simulink library "chy_framelib"  (R2016a)
settings: Solver=ode1  StartTime=0.0  StopTime=Inf  FixedStep=0.001  RelTol=1e-3
undefined symbols (not defined in the file): emot_Ri_Inv
libraries: Powernet x1, Energy_converter_Electrical_to_Mechanical x1
settings Model: Creator=ASRANJA  LastModifiedBy=KNWINDE
settings DataIOCC: LimitDataPoints=on  SaveFormat=Array  SignalLoggingSaveFormat=ModelDataLogs
settings OptimizationCC: BlockReduction=off  OptimizeBlockIOStorage=off  BufferReuse=off  GlobalBufferReuse=off  ExpressionFolding=off  ExpressionDepthLimit=2147483647  LocalBlockOutputs=off
settings DebuggingCC: UnderspecifiedInitializationDetection=Classic  MergeDetectMultiDrivingBlocksExec=none  SolverPrmCheckMsg=warning  MultiTaskDSMMsg=warning  MultiTaskCondExecSysMsg=none  StateNameClashWarn=warning  StrictBusMsg=None
settings HardwareCC: ProdBitPerPointer=32  ProdLargestAtomicFloat=None  ProdIntDivRoundTo=Undefined  ProdEndianess=Unspecified  ProdWordSize=32  ProdHWDeviceType=32-bit Generic
settings ModelReferenceCC: PropagateSignalLabelsOutOfModel=off
settings RTWCC: SystemTargetFile=rti1401.tlc  MakeCommand=make_rti  TemplateMakefile=rti1401.tmf  Description=dSPACE DS1401 Hardware Platform
settings STFCustomTargetCC: ModelReferenceCompliant=off  GeneratePreprocessorConditionals=Disable all  CombineOutputUpdateFcns=on  MatFileLogging=on  MATLABClassNameForMDSCustomization=Simulink.SoftwareTarget.TargetSpecificTriggerConfigurationBase  CPPClassGenCompliant=on  GRTInterface=off  SystemTargetFile=rti1401.tlc
settings ConfigComp: CovModelRefEnable=Off

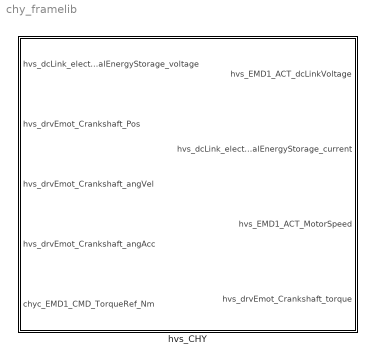
== system chy_framelib ==
  hvs_CHY : Subsystem

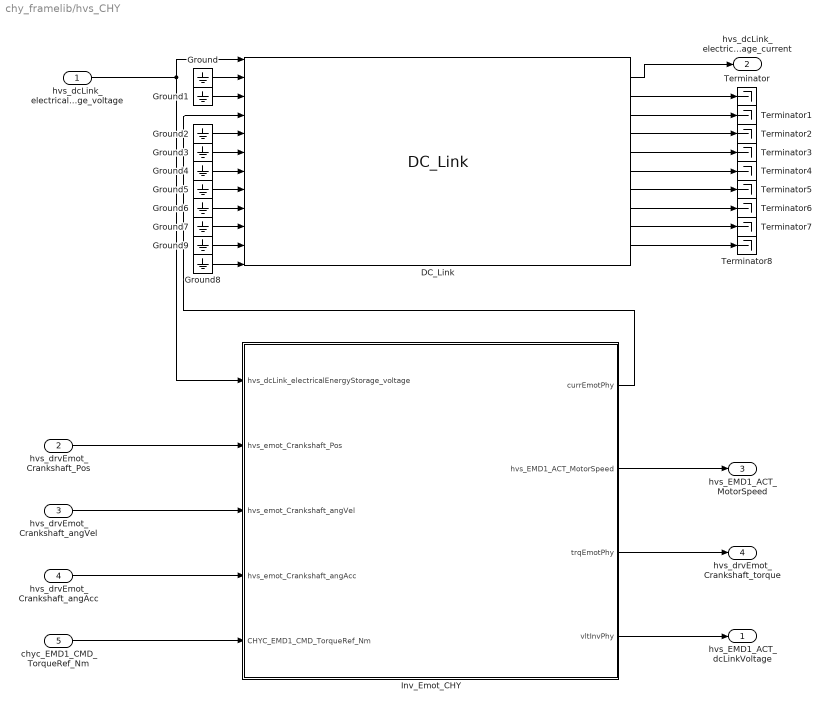
== system chy_framelib/hvs_CHY ==
  hvs_dcLink_electricalEnergyStorage_voltage : Inport
  hvs_drvEmot_Crankshaft_Pos : Inport  Port=2
  hvs_drvEmot_Crankshaft_angVel : Inport  Port=3
  hvs_drvEmot_Crankshaft_angAcc : Inport  Port=4
  chyc_EMD1_CMD_TorqueRef_Nm : Inport  Port=5
  DC_Link : Powernet/DC_Link
  Ground{,1..9} (10 alike) : Ground
  Inv_Emot_CHY : Subsystem
  Terminator{,1..8} (9 alike) : Terminator
  hvs_EMD1_ACT_dcLinkVoltage : Outport
  hvs_dcLink_electricalEnergyStorage_current : Outport  Port=2
  hvs_EMD1_ACT_MotorSpeed : Outport  Port=3
  hvs_drvEmot_Crankshaft_torque : Outport  Port=4
  wires:
  Inv_Emot_CHY/4(vltInvPhy) -> hvs_EMD1_ACT_dcLinkVoltage/1
  hvs_dcLink_electricalEnergyStorage_voltage/1 -> DC_Link/1, Inv_Emot_CHY/1(hvs_dcLink_electricalEnergyStorage_voltage)
  DC_Link/1 -> hvs_dcLink_electricalEnergyStorage_current/1
  hvs_drvEmot_Crankshaft_Pos/1 -> Inv_Emot_CHY/2(hvs_emot_Crankshaft_Pos)
  hvs_drvEmot_Crankshaft_angVel/1 -> Inv_Emot_CHY/3(hvs_emot_Crankshaft_angVel)
  hvs_drvEmot_Crankshaft_angAcc/1 -> Inv_Emot_CHY/4(hvs_emot_Crankshaft_angAcc)
  chyc_EMD1_CMD_TorqueRef_Nm/1 -> Inv_Emot_CHY/5(CHYC_EMD1_CMD_TorqueRef_Nm)
  Inv_Emot_CHY/1(currEmotPhy) -> DC_Link/4
  Ground/1 -> DC_Link/2
  Ground1/1 -> DC_Link/3
  Ground2/1 -> DC_Link/5
  Ground3/1 -> DC_Link/6
  Ground4/1 -> DC_Link/7
  DC_Link/2 -> Terminator/1
  DC_Link/3 -> Terminator1/1
  DC_Link/4 -> Terminator2/1
  DC_Link/5 -> Terminator3/1
  DC_Link/6 -> Terminator4/1
  Inv_Emot_CHY/2(hvs_EMD1_ACT_MotorSpeed) -> hvs_EMD1_ACT_MotorSpeed/1
  DC_Link/7 -> Terminator5/1
  Ground5/1 -> DC_Link/8
  Ground6/1 -> DC_Link/9
  Ground7/1 -> DC_Link/10
  Inv_Emot_CHY/3(trqEmotPhy) -> hvs_drvEmot_Crankshaft_torque/1
  Ground8/1 -> DC_Link/12
  Ground9/1 -> DC_Link/11
  DC_Link/8 -> Terminator6/1
  DC_Link/9 -> Terminator7/1
  DC_Link/10 -> Terminator8/1

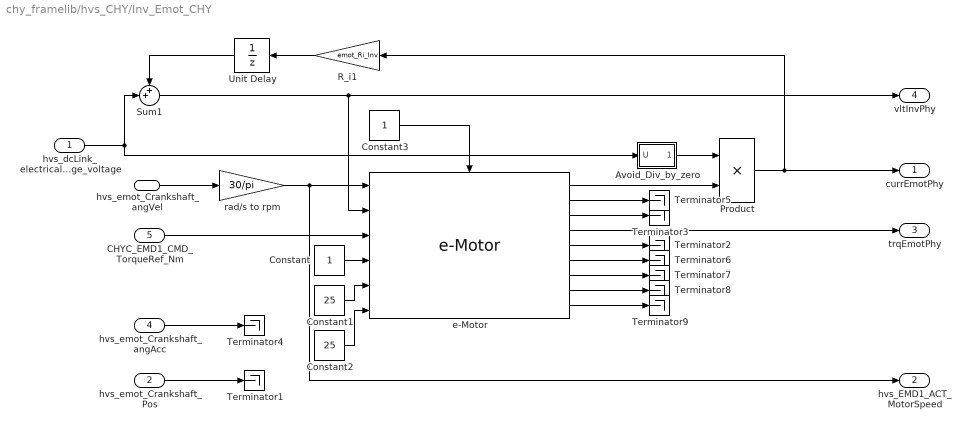
== system chy_framelib/hvs_CHY/Inv_Emot_CHY ==
  hvs_dcLink_electricalEnergyStorage_voltage : Inport
  hvs_emot_Crankshaft_Pos : Inport  Port=2
  hvs_emot_Crankshaft_angVel : Inport  Port=3
  hvs_emot_Crankshaft_angAcc : Inport  Port=4
  CHYC_EMD1_CMD_TorqueRef_Nm : Inport  Port=5
  Avoid_Div_by_zero : Subsystem
  Constant : Constant
  Constant1 : Constant  Value=25
  Constant2 : Constant  Value=25
  Constant3 : Constant
  Product : Product
  R_i1 : Gain  Gain=emot_Ri_Inv
  Sum1 : Sum  Inputs=++|
  Terminator{1..9} (9 alike) : Terminator
  Unit Delay : UnitDelay  SampleTime=-1
  e-Motor : Energy_converter_Electrical_to_Mechanical/e-Motor  SystemSampleTime=-1
  rad/s to rpm : Gain  Gain=30/pi
  currEmotPhy : Outport
  hvs_EMD1_ACT_MotorSpeed : Outport  Port=2
  trqEmotPhy : Outport  Port=3
  vltInvPhy : Outport  Port=4
  wires:
  Avoid_Div_by_zero/1(1/U) -> Product/1
  Constant/1 -> e-Motor/4
  e-Motor/1 -> Product/2
  e-Motor/4 -> trqEmotPhy/1
  hvs_emot_Crankshaft_angAcc/1 -> Terminator4/1
  hvs_emot_Crankshaft_angVel/1 -> rad/s to rpm/1
  CHYC_EMD1_CMD_TorqueRef_Nm/1 -> e-Motor/3
  hvs_emot_Crankshaft_Pos/1 -> Terminator1/1
  Product/1 -> R_i1/1, currEmotPhy/1
  hvs_dcLink_electricalEnergyStorage_voltage/1 -> Sum1/2, Avoid_Div_by_zero/1(U)
  Unit Delay/1 -> Sum1/1
  R_i1/1 -> Unit Delay/1
  Sum1/1 -> e-Motor/2, vltInvPhy/1
  rad/s to rpm/1 -> e-Motor/1, hvs_EMD1_ACT_MotorSpeed/1
  e-Motor/2 -> Terminator5/1
  e-Motor/3 -> Terminator3/1
  e-Motor/5 -> Terminator2/1
  e-Motor/6 -> Terminator6/1
  e-Motor/7 -> Terminator7/1
  e-Motor/8 -> Terminator8/1
  e-Motor/9 -> Terminator9/1
  Constant1/1 -> e-Motor/5
  Constant2/1 -> e-Motor/6
  Constant3/1 -> e-Motor/Enable

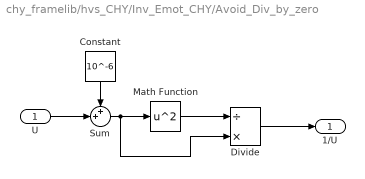
== system chy_framelib/hvs_CHY/Inv_Emot_CHY/Avoid_Div_by_zero ==
  U : Inport
  Constant : Constant  Value=10^-6
  Divide : Product  Inputs=/*
  Math Function : Math  Operator=square  SaturateOnIntegerOverflow=on
  Sum : Sum  Inputs=++|
  1/U : Outport
  wires:
  U/1 -> Sum/2
  Constant/1 -> Sum/1
  Sum/1 -> Math Function/1, Divide/2
  Math Function/1 -> Divide/1
  Divide/1 -> 1/U/1
